simulink model "TruckSuspension"  (R2020a)
settings: Solver=VariableStepAuto  StartTime=0.0  StopTime=100  RelTol=1e-3
settings Model: Creator=DELL  LastModifiedBy=DELL
settings DataIOCC: ExternalInput=[t, signal]  LoadExternalInput=on

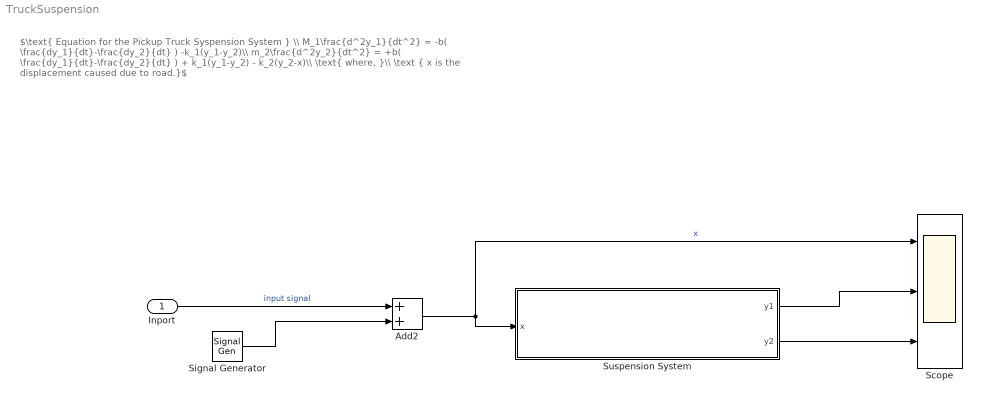
== system TruckSuspension ==
  note: $\text{ Equation for the Pickup Truck Syspension System } \\ M_1\frac{d^2y_1}{dt^2} = -b( \frac{dy_1}{dt}-\frac{dy_2}{dt} ) -k_1(y_1-y_2)\\ m_2\frac{d^2y_2}{dt^2} = +b( \frac{dy_1}{dt}-\frac{dy_2}{dt} ) + k_1(y_1-y_2) - k_2(y_2-x)\\ \text{ where, }\\ \text { x is the displacement caused due to road.}$
  Inport : Inport
  Add2 : Sum
  Scope : Scope  NumInputPorts=3
  Signal Generator : SignalGenerator  WaveForm=random  Units=rad/sec
  Suspension System : Subsystem  mask{M1=500, k1=250, b=1, m2=20, k2=1}
      mask prompts: M1 "Mass of vehicle (M1)"; k1 "Spring Constant (k1)"; b "Damper Constant (b)"; m2 "Mass of Wheel (m2)"
      mask DialogControl DescGroupVar Prompt: PickUp Truck
      mask DialogControl DescTextVar Prompt: Suspension System Parameters
      mask DialogControl Container3 Prompt: Vehicale Parameter
      mask DialogControl Container4 Prompt: Suspension Parameters
      mask DialogControl Container7 Prompt: Wheel Parameters
  wires:
  Inport/1 -> Add2/1  "input signal"
  Signal Generator/1 -> Add2/2
  Add2/1 -> Scope/1, Suspension System/1(x)  "x"
  Suspension System/1(y1) -> Scope/2
  Suspension System/2(y2) -> Scope/3

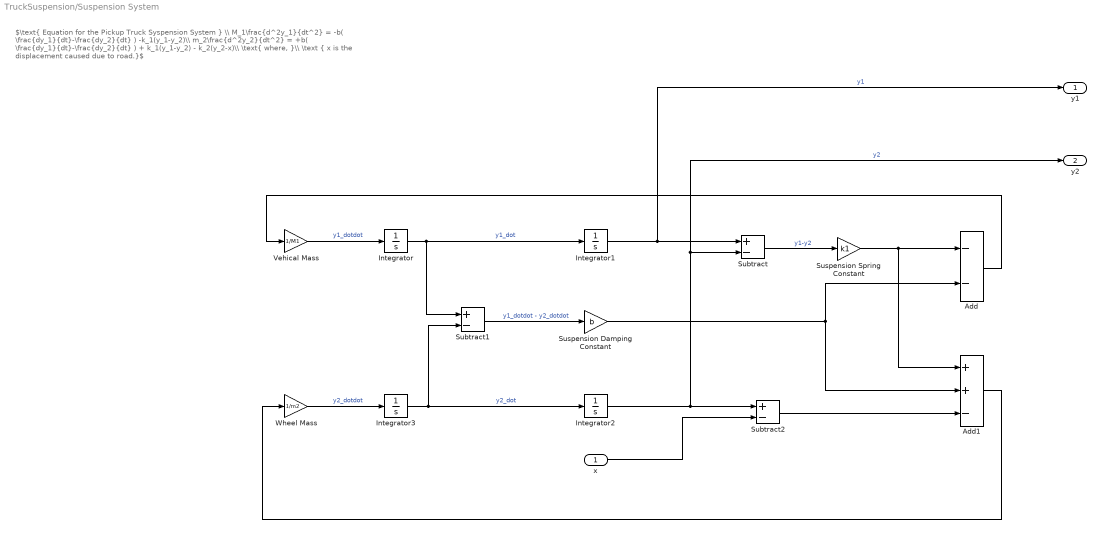
== system TruckSuspension/Suspension System ==
  note: $\text{ Equation for the Pickup Truck Syspension System } \\ M_1\frac{d^2y_1}{dt^2} = -b( \frac{dy_1}{dt}-\frac{dy_2}{dt} ) -k_1(y_1-y_2)\\ m_2\frac{d^2y_2}{dt^2} = +b( \frac{dy_1}{dt}-\frac{dy_2}{dt} ) + k_1(y_1-y_2) - k_2(y_2-x)\\ \text{ where, }\\ \text { x is the displacement caused due to road.}$
  x : Inport
  Add : Sum  Inputs=--
  Add1 : Sum  Inputs=++-
  Integrator{,1..3} (4 alike) : Integrator
  Subtract : Sum  Inputs=+-
  Subtract1 : Sum  Inputs=+-
  Subtract2 : Sum  Inputs=+-
  Suspension Damping Constant : Gain  Gain=b
  Suspension Spring Constant : Gain  Gain=k1
  Vehical Mass : Gain  Gain=1/M1
  Wheel Mass : Gain  Gain=1/m2
  y1 : Outport
  y2 : Outport  Port=2
  wires:
  Suspension Damping Constant/1 -> Add/2, Add1/2
  Subtract2/1 -> Add1/3
  Integrator/1 -> Subtract1/1, Integrator1/1  "y1_dot"
  Integrator3/1 -> Subtract1/2, Integrator2/1  "y2_dot"
  Add1/1 -> Wheel Mass/1
  Add/1 -> Vehical Mass/1
  Vehical Mass/1 -> Integrator/1  "y1_dotdot"
  Subtract1/1 -> Suspension Damping Constant/1  "y1_dotdot - y2_dotdot"
  Integrator1/1 -> y1/1, Subtract/1  "y1"
  Integrator2/1 -> y2/1, Subtract/2, Subtract2/1  "y2"
  Wheel Mass/1 -> Integrator3/1  "y2_dotdot"
  Subtract/1 -> Suspension Spring Constant/1  "y1-y2"
  Suspension Spring Constant/1 -> Add1/1, Add/1
  x/1 -> Subtract2/2
